simulink model "simulacao_test2"  (R2018a)
settings: Solver=VariableStepAuto  StartTime=0.0  StopTime=10.0  RelTol=1e-3
settings Model: Creator=LabT5  LastModifiedBy=LabT5

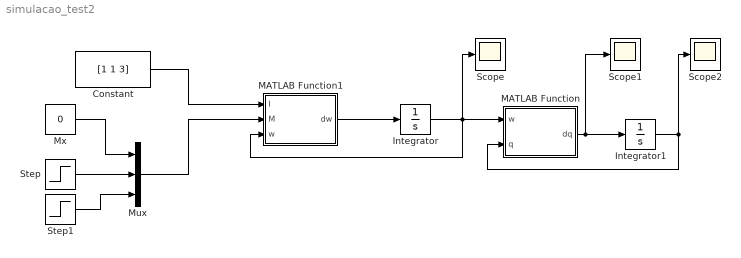
== system simulacao_test2 ==
  Constant : Constant  Value=[1 1 3]
  Integrator : Integrator  InitialCondition=[0 0 0]
  Integrator1 : Integrator  InitialCondition=[1 0 0 0]
  MATLAB Function : MATLAB Function  TreatAsAtomicUnit=on
  MATLAB Function1 : MATLAB Function  TreatAsAtomicUnit=on
  Mux : Mux  Inputs=3
  Mx : Constant  Value=0
  Scope : Scope
  Scope1 : Scope
  Scope2 : Scope
  Step : Step  Time=0.5  Before=2  After=0  SampleTime=0
  Step1 : Step  Before=1  After=0  SampleTime=0
  wires:
  Mx/1 -> Mux/1
  Constant/1 -> MATLAB Function1/1(I)
  Step1/1 -> Mux/3
  Step/1 -> Mux/2
  MATLAB Function1/1(dw) -> Integrator/1
  Integrator/1 -> Scope/1, MATLAB Function1/3(w), MATLAB Function/1(w)
  MATLAB Function/1(dq) -> Scope1/1, Integrator1/1
  Mux/1 -> MATLAB Function1/2(M)
  Integrator1/1 -> MATLAB Function/2(q), Scope2/1

== matlab function simulacao_test2/MATLAB Function1 ==
  data: I input; dw output; M input; w input
function dw = Eq_Euler(I,M,w)
wx = w(1);
wy = w(2);
wz = w(3);
Ix = I(1);
Iy = I(2);
Iz = I(3);

Mx = M(1);
My = M(2);
Mz = M(3);

dwx = (Mx - wy*wz*(Iz - Iy))/Ix;
dwy = (My - wx*wz*(Ix - Iz))/Iy;
dwz = (Mz - wx*wy*(Iy - Ix))/Iz;

dw=[dwx dwy dwz]';

== matlab function simulacao_test2/MATLAB Function ==
  data: w input; dq output; q input
function dq = cinematica(w,q)

wx = w(1);
wy = w(2);
wz = w(3);

q = q/norm(q);
qteta = q(1);
qx = q(2);
qy = q(3);
qz = q(4);

W = [0 -wx -wy -wz; wx 0 wz -wy; wy -wz 0 wx; wz wy -wx 0];
dq=0.5*W*[qteta qx qy qz]';
